simulink model "parameters_identification"  (R2024a)
settings: Solver=VariableStepAuto  StartTime=0.0  StopTime=5  RelTol=1e-3
values from neighbouring files (symbols this model uses):
  f = (1-phi_m)/gamma_m    [electrical_mechanical_parameters.m]
  J = -(f*h)/log(phi_m)    [electrical_mechanical_parameters.m]
  Ka = Kg    [electrical_mechanical_parameters.m]
  Kg = Kt*(w'*e)/(w'*w)    [computing_Kg.m]    (also in electrical_mechanical_parameters.m = Kg)
  La = -(Ra*h)/log(phi_e)    [electrical_mechanical_parameters.m]
  Ra = (1-phi_e)/gamma_e    [electrical_mechanical_parameters.m]
undefined symbols (not defined in the file or in its folder): Kt
settings Model: Creator=Guilherme  LastModifiedBy=Guilherme

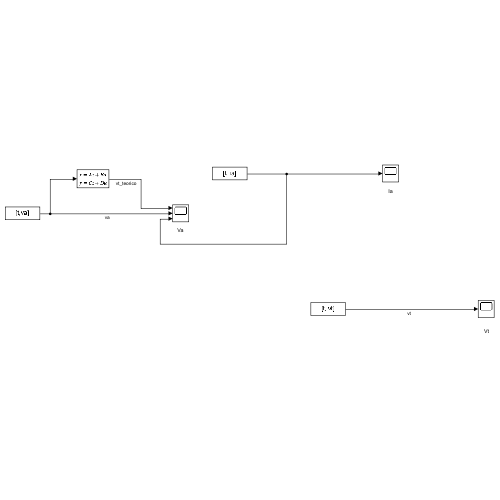
[thumbnail: Simulink's stored preview of the top-level diagram]
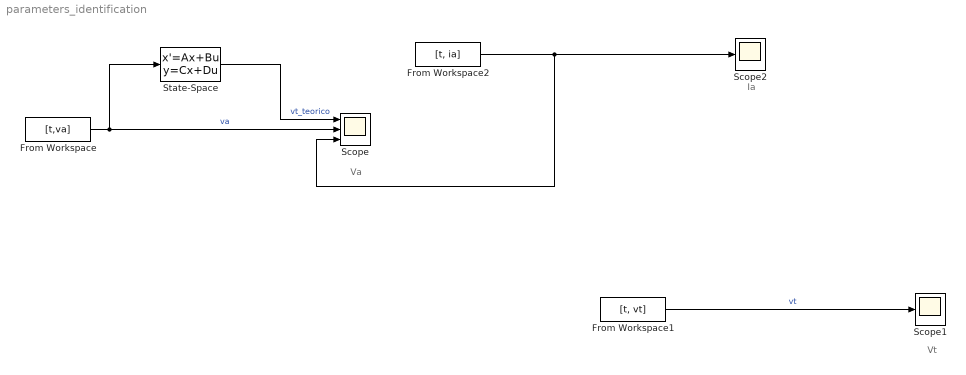
== system parameters_identification ==
  note: Ia
  note: Va
  note: Vt
  From Workspace : FromWorkspace  VariableName=[t,va]
  From Workspace1 : FromWorkspace  VariableName=[t, vt]
  From Workspace2 : FromWorkspace  VariableName=[t, ia]
  Scope : Scope  NumInputPorts=3
  Scope1 : Scope
  Scope2 : Scope
  State-Space : StateSpace  A=[-Ra/La, -Kg/(Kt*La); (Ka*Kt)/J, -f/J]  B=[1/La; 0]  C=[1, 0]  D=[0]  InitialCondition=0
  wires:
  From Workspace/1 -> State-Space/1, Scope/2  "va"
  From Workspace1/1 -> Scope1/1  "vt"
  From Workspace2/1 -> Scope/3, Scope2/1
  State-Space/1 -> Scope/1  "vt_teorico"
